simulink model "filter_block_test"  (R2021b)
settings: Solver=VariableStepAuto  StartTime=0.0  StopTime=stop_time-1  RelTol=1e-3
libraries: dspsrcs4 x2
settings Model: Creator=torha  LastModifiedBy=torha

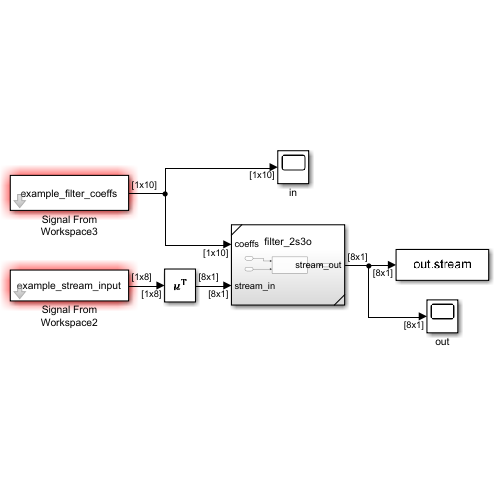
[thumbnail: Simulink's stored preview of the top-level diagram]
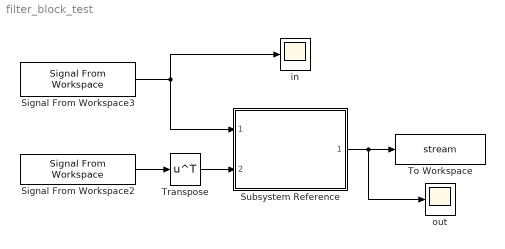
== system filter_block_test ==
  Signal From Workspace2 : dspsrcs4/Signal From Workspace  X=example_stream_input  Ts=1  nsamps=1  OutputAfterFinalValue=Setting to zero  ignoreOrWarnInputAndFrameLengths=off  OutputFrames=off
  Signal From Workspace3 : dspsrcs4/Signal From Workspace  X=example_filter_coeffs  Ts=1  nsamps=1  OutputAfterFinalValue=Setting to zero  ignoreOrWarnInputAndFrameLengths=off  OutputFrames=off
  Subsystem Reference : Subsystem  ReferencedSubsystem=filter_2s3o
  To Workspace : ToWorkspace  VariableName=stream  SampleTime=-1
      settings: Save2DSignal=2-D array (concatenate along first dimension)
  Transpose : Math  Operator=transpose  SaturateOnIntegerOverflow=on
  in : Scope
  out : Scope
  wires:
  Signal From Workspace3/1 -> Subsystem Reference/1, in/1
  Signal From Workspace2/1 -> Transpose/1
  Subsystem Reference/1 -> out/1, To Workspace/1
  Transpose/1 -> Subsystem Reference/2
